simulink model "Simulink_san"  (R2019b)
settings: Solver=VariableStepAuto  StartTime=0.0  StopTime=100  RelTol=1e-3
values from neighbouring files (symbols this model uses):
  K = lqr(A_subs,B_subs',Q,R)    [Inverted_pendulum.m]
settings Model: Creator=2020  LastModifiedBy=divya

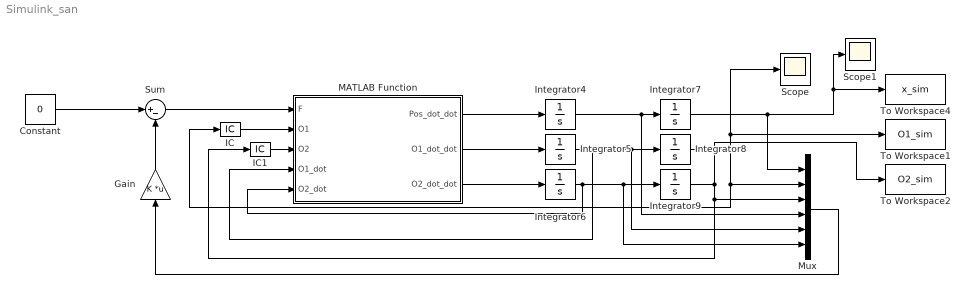
== system Simulink_san ==
  Constant : Constant  Value=0
  Gain : Gain  Gain=K  Multiplication=Matrix(K*u)
  IC : InitialCondition  Value=pi/10
  IC1 : InitialCondition  Value=pi/20
  Integrator{4..9} (6 alike) : Integrator
  MATLAB Function : MATLAB Function  TreatAsAtomicUnit=on
  Mux : Mux  Inputs=6
  Scope : Scope
  Scope1 : Scope
  Sum : Sum  Inputs=|+-
  To Workspace1 : ToWorkspace  VariableName=O1_sim  SampleTime=-1
      settings: Save2DSignal=2-D array (concatenate along first dimension)
  To Workspace2 : ToWorkspace  VariableName=O2_sim  SampleTime=-1
      settings: Save2DSignal=2-D array (concatenate along first dimension)
  To Workspace4 : ToWorkspace  VariableName=x_sim  SampleTime=-1
      settings: Save2DSignal=2-D array (concatenate along first dimension)
  wires:
  Constant/1 -> Sum/1
  Sum/1 -> MATLAB Function/1(F)
  MATLAB Function/1(Pos_dot_dot) -> Integrator4/1
  MATLAB Function/2(O1_dot_dot) -> Integrator5/1
  MATLAB Function/3(O2_dot_dot) -> Integrator6/1
  Integrator4/1 -> Mux/4, Integrator7/1
  Integrator6/1 -> Mux/6, Integrator9/1, MATLAB Function/5(O2_dot)
  Integrator5/1 -> Mux/5, Integrator8/1, MATLAB Function/4(O1_dot)
  Integrator9/1 -> To Workspace2/1, IC1/1, Mux/3
  Integrator8/1 -> To Workspace1/1, Scope/1, IC/1, Mux/2
  Integrator7/1 -> Mux/1, To Workspace4/1, Scope1/1
  Mux/1 -> Gain/1
  Gain/1 -> Sum/2
  IC/1 -> MATLAB Function/2(O1)
  IC1/1 -> MATLAB Function/3(O2)

== matlab function Simulink_san/MATLAB Function ==
  data: F input; Pos_dot_dot output; O1 input; O2 input; O1_dot input; O2_dot input; O1_dot_dot output; O2_dot_dot output
function [Pos_dot_dot,O1_dot_dot,O2_dot_dot] = output(F,O1,O2,O1_dot,O2_dot)

M = 1000;
m1 = 100;
m2 = 100;
L1 = 20;
L2 = 10;
g = 10;


% num = F- m1*g*sin(O1)*cos(O1)- m2*g*sin(O2)*cos(O2)- m1*L1*(O1_dot^2)*sin(O1)- m2*L2*(O2_dot^2)*sin(O2);
% den = (M+m1+m2) - m1*(cos(O1))^2 - m2*(cos(O2))^2;
% Pos_dot_dot = num/den;
% 
% O1_dot_dot= (Pos_dot_dot*cos(O1)-g*sin(O1))/L1;
% 
% O2_dot_dot= (Pos_dot_dot*cos(O2)-g*sin(O2))/L2;


Pos_dot_dot = -(L1*m1*sin(O1)*O1_dot^2 - F + L2*m2*sin(O2)*O2_dot^2 + g*m1*cos(O1)*sin(O1) + g*m2*cos(O2)*sin(O2))/(- m1*cos(O1)^2 - m2*cos(O2)^2 + M + m1 + m2);
 
O1_dot_dot = -(g*sin(O1) + (cos(O1)*(L1*m1*sin(O1)*O1_dot^2 - F + L2*m2*sin(O2)*O2_dot^2 + g*m1*cos(O1)*sin(O1) + g*m2*cos(O2)*sin(O2)))/(- m1*cos(O1)^2 - m2*cos(O2)^2 + M + m1 + m2))/L1;
 
O2_dot_dot = -(g*sin(O2) + (cos(O2)*(L1*m1*sin(O1)*O1_dot^2 - F + L2*m2*sin(O2)*O2_dot^2 + g*m1*cos(O1)*sin(O1) + g*m2*cos(O2)*sin(O2)))/(- m1*cos(O1)^2 - m2*cos(O2)^2 + M + m1 + m2))/L2;
